simulink model "experiment_supervisor"  (R2023b)
settings: Solver=FixedStepDiscrete  StartTime=0.0  StopTime=inf  FixedStep=Ts  RelTol=1e-3
model workspace (MAT data in the model file):
  Ts = Simulink.Parameter
  Ts.Value = 0.01
  Ts.DataType = 'auto'
  Ts.DocUnits = 's'
  Ts.Complexity = 'real'
  Ts.Dimensions = [1 1]
  board_ID = Simulink.Parameter
  board_ID.Value = 1
  board_ID.DataType = 'auto'
  board_ID.Complexity = 'real'
  board_ID.Dimensions = [1 1]
undefined symbols (not defined in the file): CAN_ANGLE_DEG2ICUB, CAN_ANGLE_ICUB2DEG, CAN_VOLT_REF_SHIFT, canChannel
libraries: canmsglib x12, canlib x4, simulink x1, hdlsllib x1
settings Model: DataDictionary=EmbeddedBoardDD.sldd  Creator=upattacini  LastModifiedBy=mfussi
settings SolverCC: AlgebraicLoopSolver=TrustRegion  DecoupledContinuousIntegration=on  MinimalZcImpactIntegration=on
settings OptimizationCC: ReuseModelBlockBuffer=off  SimCompilerOptimization=on
settings DebuggingCC: ParameterPrecisionLossMsg=none  UnconnectedInputMsg=warning  UnconnectedOutputMsg=warning  UnconnectedLineMsg=warning  ArithmeticOperatorsInVariantConditions=warning
settings HardwareCC: ProdBitPerLong=64  ProdHWDeviceType=Intel->x86-64 (Linux 64)
settings ModelReferenceCC: EnableRefExpFcnMdlSchedulingChecks=on
settings SFSimCC: SimUseLocalCustomCode=off  CustomCodeUndefinedFunction=UseInterfaceOnly
settings RTWCC: Description=Simulink Desktop Real-Time  SystemTargetFile=sldrt.tlc  TemplateMakefile=sldrt.tmf  RTWUseLocalCustomCode=off  RTWCompilerOptimization=on  DLArmComputeVersion=19.05
settings CodeAppCC: MaxIdLength=95
settings SimulinkDesktopRealTimeCC: TargetLibSuffix=_sldrt.a  TargetPreCompLibLocation=C:\Program Files\MATLAB\R2023b\toolbox\sldrt\lib\win64

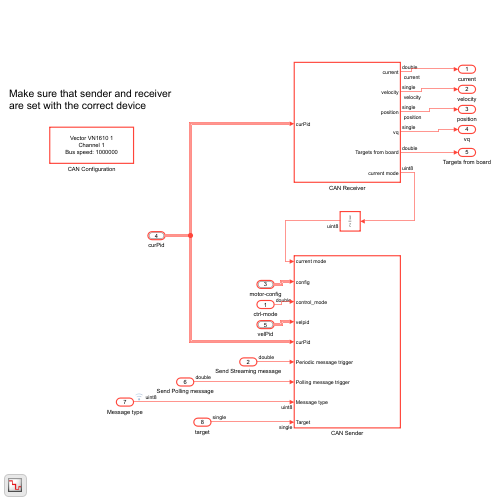
[thumbnail: Simulink's stored preview of the top-level diagram]
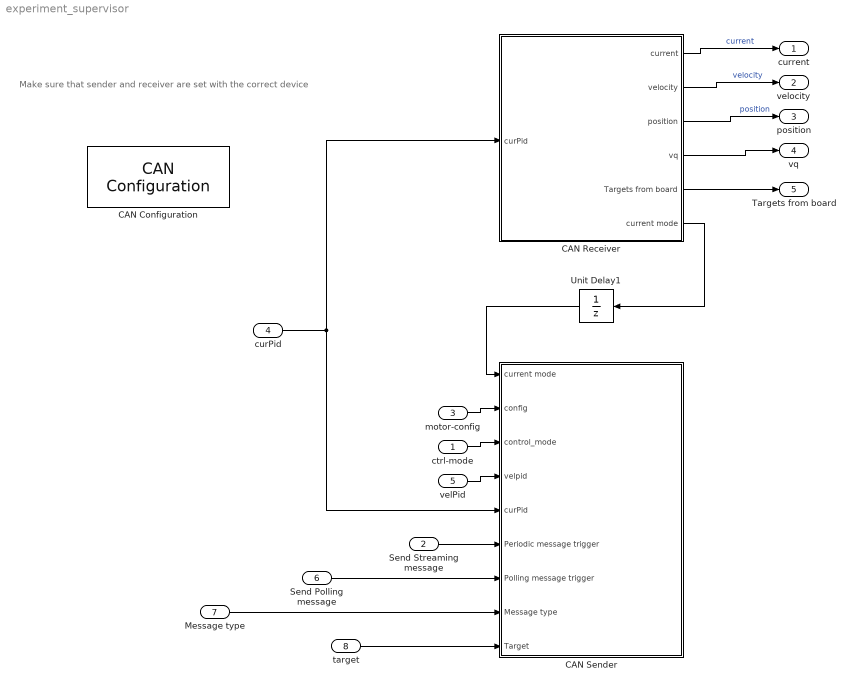
== system experiment_supervisor ==
  note: Make sure that sender and receiver
      | are set with the correct device
  ctrl-mode : Inport
  Send Streaming message : Inport  Port=2
  motor-config : Inport  Port=3  OutDataTypeStr=Bus: MotorConfig
  curPid : Inport  Port=4  OutDataTypeStr=Bus: PIDConfig
  velPid : Inport  Port=5  OutDataTypeStr=Bus: PIDConfig
  Send Polling message : Inport  Port=6
  Message type : Inport  Port=7
  target : Inport  Port=8  OutDataTypeStr=single
  CAN Configuration : canlib/CAN Configuration  BlockHandle=989.0002  Device=Vector VN1610 1 (Channel 1)  DeviceMenu=Vector VN1610 1 (Channel 1)  ObjConstructor=canChannel('Vector', 'VN1610 1', 1)  BusSpeed=1000000  EnableBitParameters=off  SJW=1  TSEG1=4  TSEG2=3  NSamples=1  AckMode=Normal
  CAN Receiver : Subsystem
  CAN Sender : Subsystem
  Unit Delay1 : UnitDelay  SampleTime=-1  HasFrameUpgradeWarning=on
  current : Outport
  velocity : Outport  Port=2
  position : Outport  Port=3
  vq : Outport  Port=4
  Targets from board : Outport  Port=5
  wires:
  CAN Receiver/6(current mode) -> Unit Delay1/1
  curPid/1 -> CAN Sender/5(curPid), CAN Receiver/1(curPid)
  CAN Receiver/5(Targets from board) -> Targets from board/1
  CAN Receiver/1(current) -> current/1  "current"
  CAN Receiver/4(vq) -> vq/1
  CAN Receiver/3(position) -> position/1  "position"
  CAN Receiver/2(velocity) -> velocity/1  "velocity"
  motor-config/1 -> CAN Sender/2(config)
  ctrl-mode/1 -> CAN Sender/3(control_mode)
  velPid/1 -> CAN Sender/4(velpid)
  Send Streaming message/1 -> CAN Sender/6(Periodic message trigger)
  Unit Delay1/1 -> CAN Sender/1(current mode)
  Send Polling message/1 -> CAN Sender/7(Polling message trigger)
  Message type/1 -> CAN Sender/8(Message type)
  target/1 -> CAN Sender/9(Target)

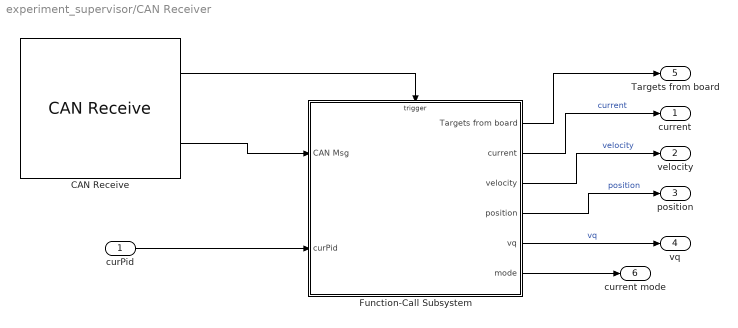
== system experiment_supervisor/CAN Receiver ==
  curPid : Inport  OutDataTypeStr=Bus: PIDConfig
  CAN Receive : canlib/CAN Receive  BlockHandle=992.0002  Device=Vector VN1610 1 (Channel 1)  DeviceMenu=Vector VN1610 1 (Channel 1)  ObjConstructor=canChannel('Vector', 'VN1610 1', 1)  EnableStandardIDsFilter=off  StdIDsCombo=Allow all  StandardIDs=0  EnableExtendedIDsFilter=off  ExtIDsCombo=Allow all  ExtendedIDs=0  SampleTime=Ts  MsgsPerTimestep=all  InternalFilterUpdateStatus=on  BusOutput=on
  Function-Call Subsystem : Subsystem  TreatAsAtomicUnit=on
  current : Outport
  velocity : Outport  Port=2
  position : Outport  Port=3
  vq : Outport  Port=4
  Targets from board : Outport  Port=5
  current mode : Outport  Port=6
  wires:
  CAN Receive/1 -> Function-Call Subsystem/Trigger
  CAN Receive/2 -> Function-Call Subsystem/1(CAN Msg)
  Function-Call Subsystem/2(current) -> current/1  "current"
  Function-Call Subsystem/3(velocity) -> velocity/1  "velocity"
  Function-Call Subsystem/4(position) -> position/1  "position"
  Function-Call Subsystem/5(vq) -> vq/1  "vq"
  Function-Call Subsystem/1(Targets from board) -> Targets from board/1
  curPid/1 -> Function-Call Subsystem/2(curPid)
  Function-Call Subsystem/6(mode) -> current mode/1

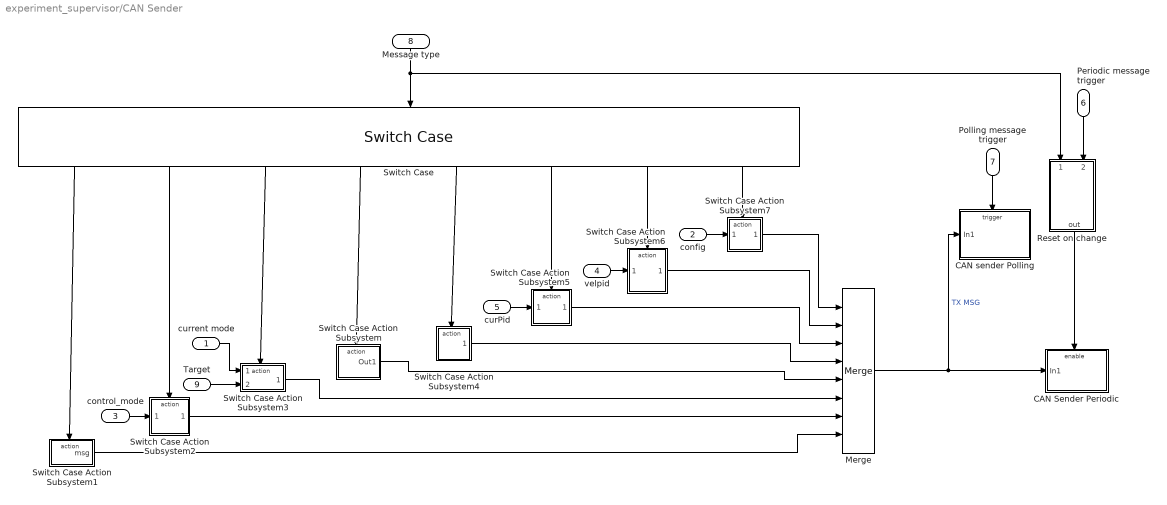
== system experiment_supervisor/CAN Sender ==
  current mode : Inport
  config : Inport  Port=2  OutDataTypeStr=Bus: MotorConfig
  control_mode : Inport  Port=3
  velpid : Inport  Port=4
  curPid : Inport  Port=5
  Periodic message trigger : Inport  Port=6
  Polling message trigger : Inport  Port=7
  Message type : Inport  Port=8  OutDataTypeStr=uint8
  Target : Inport  Port=9  OutDataTypeStr=single
  CAN Sender Periodic : Subsystem  TreatAsAtomicUnit=on
  CAN sender Polling : Subsystem
  Merge : Merge  Inputs=8
  Reset on change : Subsystem
  Switch Case : SwitchCase  CaseConditions={1,2,3,4,5,6,7,8}  ShowDefaultCase=off
  Switch Case Action Subsystem : Subsystem  TreatAsAtomicUnit=on
  Switch Case Action Subsystem1 : Subsystem  TreatAsAtomicUnit=on
  Switch Case Action Subsystem2 : Subsystem  TreatAsAtomicUnit=on
  Switch Case Action Subsystem3 : Subsystem  TreatAsAtomicUnit=on
  Switch Case Action Subsystem4 : Subsystem  TreatAsAtomicUnit=on
  Switch Case Action Subsystem5 : Subsystem  TreatAsAtomicUnit=on
  Switch Case Action Subsystem6 : Subsystem  TreatAsAtomicUnit=on
  Switch Case Action Subsystem7 : Subsystem  TreatAsAtomicUnit=on
  wires:
  Message type/1 -> Reset on change/1(message type), Switch Case/1
  Polling message trigger/1 -> CAN sender Polling/Trigger
  Merge/1 -> CAN Sender Periodic/1(In1), CAN sender Polling/1(In1)  "TX MSG"
  control_mode/1 -> Switch Case Action Subsystem2/1(control_mode)
  current mode/1 -> Switch Case Action Subsystem3/1(mode)
  Target/1 -> Switch Case Action Subsystem3/2(target)
  Switch Case/1 -> Switch Case Action Subsystem1/Action
  Switch Case/2 -> Switch Case Action Subsystem2/Action
  Switch Case/3 -> Switch Case Action Subsystem3/Action
  Switch Case/4 -> Switch Case Action Subsystem/Action
  Switch Case/5 -> Switch Case Action Subsystem4/Action
  Switch Case/6 -> Switch Case Action Subsystem5/Action
  Switch Case/7 -> Switch Case Action Subsystem6/Action
  Switch Case/8 -> Switch Case Action Subsystem7/Action
  config/1 -> Switch Case Action Subsystem7/1(cfg)
  Switch Case Action Subsystem7/1(Out1) -> Merge/1
  Switch Case Action Subsystem6/1(Out1) -> Merge/2
  Switch Case Action Subsystem5/1(" ") -> Merge/3
  Switch Case Action Subsystem4/1(Out1) -> Merge/4
  Switch Case Action Subsystem/1(Out1) -> Merge/5
  Switch Case Action Subsystem3/1(msg) -> Merge/6
  Switch Case Action Subsystem2/1(msg) -> Merge/7
  Switch Case Action Subsystem1/1(msg) -> Merge/8
  curPid/1 -> Switch Case Action Subsystem5/1(curPid)
  velpid/1 -> Switch Case Action Subsystem6/1(velPid1)
  Periodic message trigger/1 -> Reset on change/2(enable periodic)
  Reset on change/1(out) -> CAN Sender Periodic/Enable

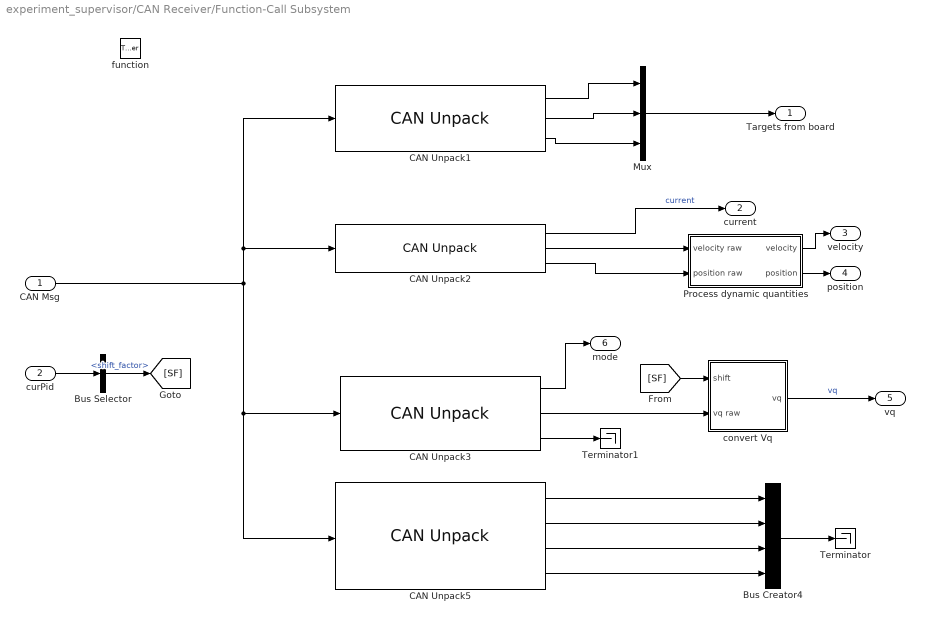
== system experiment_supervisor/CAN Receiver/Function-Call Subsystem ==
  CAN Msg : Inport
  curPid : Inport  Port=2  OutDataTypeStr=Bus: PIDConfig
  function : TriggerPort  TriggerType=function-call  VariantControl=(inherit)
  Bus Creator4 : BusCreator  Inputs=4
  Bus Selector : BusSelector  OutputSignals=shift_factor
  CAN Unpack1 : canmsglib/CAN Unpack  MsgList=(none)  MsgName=TARGETS  MsgIDType=Standard (11-bit identifier)  MsgIdentifier=0x10F  MsgLength=8  SignalInfo={ 'Target1', '0', '16', 'LE', 'signed', 'Standard', '0', '1', '0', '-Inf', 'Inf'; 'Target2', '16', '16', 'LE', 'signed', 'Standard', '0', '1', '0', '-Inf', 'Inf'; 'Target3', '32', '16', 'LE', 'signed', 'Standard', '0', '1', '0', '-Inf', 'Inf' }  IDPort=off  TimestampPort=off  ErrorPort=off  RemotePort=off  LengthPort=off  StatusPort=off  ApplyMinMax=off
  CAN Unpack2 : canmsglib/CAN Unpack  MsgList=(none)  MsgName=FOC  MsgIDType=Standard (11-bit identifier)  MsgIdentifier=0x110  MsgLength=8  SignalInfo={ 'current', '0', '16', 'LE', 'signed', 'Standard', '0', '1', '0', '-Inf', 'Inf'; 'velocity', '16', '16', 'LE', 'signed', 'Standard', '0', '1', '0', '-Inf', 'Inf'; 'position', '32', '32', 'LE', 'signed', 'Standard', '0', '1', '0', '-Inf', 'Inf' }  IDPort=off  TimestampPort=off  ErrorPort=off  RemotePort=off  LengthPort=off  StatusPort=off  ApplyMinMax=off
  CAN Unpack3 : canmsglib/CAN Unpack  MsgList=(none)  MsgName=STATUS  MsgIDType=Standard (11-bit identifier)  MsgIdentifier=0x113  MsgLength=8  SignalInfo={ 'mode', '0', '8', 'LE', 'unsigned', 'Standard', '0', '1', '0', '-Inf', 'Inf'; 'pwm', '16', '16', 'LE', 'signed', 'Standard', '0', '1', '0', '-Inf', 'Inf'; 'fault', '32', '8', 'LE', 'unsigned', 'Standard', '0', '1', '0', '-Inf', 'Inf' }  IDPort=off  TimestampPort=off  ErrorPort=off  RemotePort=off  LengthPort=off  StatusPort=off  ApplyMinMax=off
  CAN Unpack5 : canmsglib/CAN Unpack  MsgList=(none)  MsgName=DISCOVER  MsgIDType=Standard (11-bit identifier)  MsgIdentifier=0x710  MsgLength=5  SignalInfo={}  IDPort=on  TimestampPort=on  ErrorPort=off  RemotePort=off  LengthPort=on  StatusPort=off  ApplyMinMax=off
      settings: DataFormat=raw data
  Mux : Mux  Inputs=3
  Process dynamic quantities : Subsystem
  Terminator : Terminator
  Terminator1 : Terminator
  convert Vq : Subsystem
  Targets from board : Outport
  current : Outport  Port=2  Unit=mA
  velocity : Outport  Port=3
  position : Outport  Port=4
  vq : Outport  Port=5  PortDimensions=1
  mode : Outport  Port=6  OutDataTypeStr=uint8
  wires:
  CAN Unpack5/4 -> Bus Creator4/4
  CAN Unpack5/3 -> Bus Creator4/3
  CAN Unpack5/2 -> Bus Creator4/2
  CAN Unpack5/1 -> Bus Creator4/1
  Bus Creator4/1 -> Terminator/1
  CAN Unpack1/1 -> Mux/1
  CAN Unpack1/2 -> Mux/2
  CAN Unpack1/3 -> Mux/3
  Mux/1 -> Targets from board/1
  curPid/1 -> Bus Selector/1
  CAN Unpack2/2 -> Process dynamic quantities/1(velocity raw)
  CAN Unpack2/1 -> current/1  "current"
  Process dynamic quantities/2(position) -> position/1
  Process dynamic quantities/1(velocity) -> velocity/1
  CAN Unpack2/3 -> Process dynamic quantities/2(position raw)
  CAN Unpack3/2 -> convert Vq/2(vq raw)
  CAN Unpack3/1 -> mode/1
  convert Vq/1(vq) -> vq/1  "vq"
  CAN Msg/1 -> CAN Unpack2/1, CAN Unpack1/1, CAN Unpack5/1, CAN Unpack3/1
  CAN Unpack3/3 -> Terminator1/1
  Bus Selector/1 -> [SF]  "<shift_factor>"
  [SF] -> convert Vq/1(shift)

== system experiment_supervisor/CAN Sender/CAN Sender Periodic ==
  In1 : Inport
  Enable : EnablePort
  CAN Transmit : canlib/CAN Transmit  BlockHandle=1101.0002  Device=Vector VN1610 1 (Channel 1)  DeviceMenu=Vector VN1610 1 (Channel 1)  ObjConstructor=canChannel('Vector', 'VN1610 1', 1)  EnableEventTransmit=off  EnablePeriodicTransmit=on  MessagePeriod=Ts
  wires:
  In1/1 -> CAN Transmit/1

== system experiment_supervisor/CAN Sender/CAN sender Polling ==
  In1 : Inport
  Trigger : TriggerPort  VariantControl=(inherit)  PortDimensions=1
  CAN Transmit : canlib/CAN Transmit  BlockHandle=1106.0002  Device=Vector VN1610 1 (Channel 1)  DeviceMenu=Vector VN1610 1 (Channel 1)  ObjConstructor=canChannel('Vector', 'VN1610 1', 1)  EnableEventTransmit=off  EnablePeriodicTransmit=off  MessagePeriod=1.000
  wires:
  In1/1 -> CAN Transmit/1

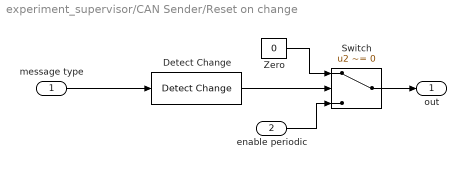
== system experiment_supervisor/CAN Sender/Reset on change ==
  message type : Inport
  enable periodic : Inport  Port=2
  Detect Change : simulink/Logic and Bit Operations/Detect Change  vinit=0  OutDataTypeStr=boolean
  Switch : Switch  Criteria=u2 ~= 0  SaturateOnIntegerOverflow=off  InputSameDT=off
  Zero : Constant  Value=0  OutDataTypeStr=Inherit: Inherit via back propagation
  out : Outport
  wires:
  Switch/1 -> out/1
  enable periodic/1 -> Switch/3
  Detect Change/1 -> Switch/2
  message type/1 -> Detect Change/1
  Zero/1 -> Switch/1

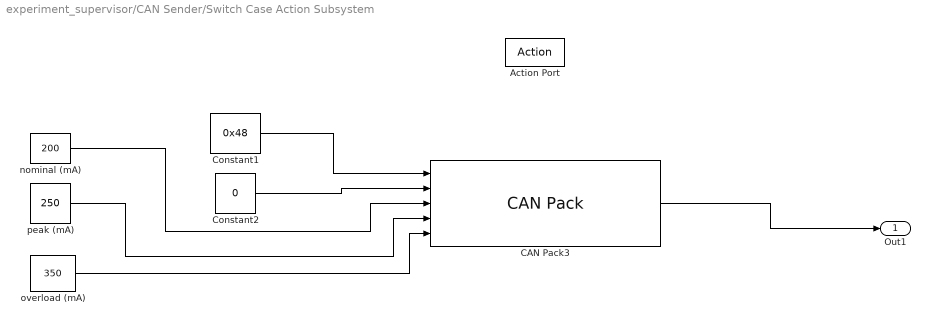
== system experiment_supervisor/CAN Sender/Switch Case Action Subsystem ==
  Action Port : ActionPort  ActionPortLabel=case [ 4 ]:
  CAN Pack3 : canmsglib/CAN Pack  MsgList=(none)  MsgName=CAN Limits  MsgIDType=Standard (11-bit identifier)  MsgIdentifier=board_ID  MsgLength=8  Remote=off  ApplyMinMax=off  BusOutput=on  SignalInfo={ 'CMD', '0', '8', 'LE', 'unsigned', 'Standard', '0', '1', '0', '-Inf', 'Inf'; 'X', '8', '8', 'LE', 'unsigned', 'Standard', '0', '1', '0', '-Inf', 'Inf'; 'NOMINAL', '16', '16', 'LE', 'unsigned', 'Standard', '0', '1', '0', '-Inf', 'Inf'; 'PEAK', '32', '16', 'LE', 'unsigned', 'Standard', '0', '1', '0', '-Inf', 'Inf'; 'OVERLOAD', '48', '16', 'LE', 'unsigned', 'Standard', '0', '1', '0', '-Inf', 'Inf' }
      settings: DataFormat=manually specified signals
  Constant1 : Constant  Value=0x48  OutDataTypeStr=Inherit: Inherit via back propagation
  Constant2 : Constant  Value=0  OutDataTypeStr=Inherit: Inherit via back propagation
  nominal (mA) : Constant  Value=200  OutDataTypeStr=Inherit: Inherit via back propagation
  overload (mA) : Constant  Value=350  OutDataTypeStr=Inherit: Inherit via back propagation
  peak (mA) : Constant  Value=250  OutDataTypeStr=Inherit: Inherit via back propagation
  Out1 : Outport
  wires:
  peak (mA)/1 -> CAN Pack3/4
  nominal (mA)/1 -> CAN Pack3/3
  overload (mA)/1 -> CAN Pack3/5
  Constant2/1 -> CAN Pack3/2
  Constant1/1 -> CAN Pack3/1
  CAN Pack3/1 -> Out1/1

== system experiment_supervisor/CAN Sender/Switch Case Action Subsystem1 ==
  Action Port : ActionPort  ActionPortLabel=case [ 1 ]:
  CAN Pack : canmsglib/CAN Pack  MsgList=(none)  MsgName=CAN Idle  MsgIDType=Standard (11-bit identifier)  MsgIdentifier=board_ID  MsgLength=2  Remote=off  ApplyMinMax=off  BusOutput=on  SignalInfo={ 'Idle', '0', '16', 'LE', 'unsigned', 'Standard', '0', '1', '0', '-Inf', 'Inf' }
      settings: DataFormat=manually specified signals
  idle-mode : Constant  Value=0x09  OutDataTypeStr=uint8
  msg : Outport
  wires:
  CAN Pack/1 -> msg/1
  idle-mode/1 -> CAN Pack/1

== system experiment_supervisor/CAN Sender/Switch Case Action Subsystem2 ==
  control_mode : Inport
  Action Port : ActionPort  ActionPortLabel=case [ 2 ]:
  CAN Pack1 : canmsglib/CAN Pack  MsgList=(none)  MsgName=SET Control Mode  MsgIDType=Standard (11-bit identifier)  MsgIdentifier=board_ID  MsgLength=2  Remote=off  ApplyMinMax=off  BusOutput=on  SignalInfo={ 'CMD', '0', '8', 'LE', 'unsigned', 'Standard', '0', '1', '0', '-Inf', 'Inf'; 'CTRL', '8', '8', 'LE', 'signed', 'Standard', '0', '1', '0', '-Inf', 'Inf' }
      settings: DataFormat=manually specified signals
  current-mode : Constant  Value=0x09  OutDataTypeStr=uint8
  msg : Outport
  wires:
  CAN Pack1/1 -> msg/1
  current-mode/1 -> CAN Pack1/1
  control_mode/1 -> CAN Pack1/2

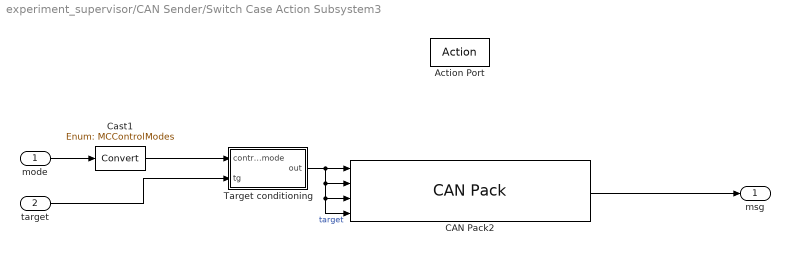
== system experiment_supervisor/CAN Sender/Switch Case Action Subsystem3 ==
  mode : Inport
  target : Inport  Port=2
  Action Port : ActionPort  ActionPortLabel=case [ 3 ]:
  CAN Pack2 : canmsglib/CAN Pack  MsgList=(none)  MsgName=CAN Target  MsgIDType=Standard (11-bit identifier)  MsgIdentifier=0x10F  MsgLength=8  Remote=off  ApplyMinMax=off  BusOutput=on  SignalInfo={ 'Target 1', '0', '16', 'LE', 'signed', 'Standard', '0', '1', '0', '-Inf', 'Inf'; 'Target 2', '16', '16', 'LE', 'signed', 'Standard', '0', '1', '0', '-Inf', 'Inf'; 'Target 3', '32', '16', 'LE', 'signed', 'Standard', '0', '1', '0', '-Inf', 'Inf'; 'Target 4', '48', '16', 'LE', 'signed', 'Standard', '0', '1', '0', '-Inf', 'Inf' }
      settings: DataFormat=manually specified signals
  Cast1 : DataTypeConversion  OutDataTypeStr=Enum: MCControlModes  SaturateOnIntegerOverflow=off  RndMeth=Floor
  Target conditioning : Subsystem
  msg : Outport
  wires:
  CAN Pack2/1 -> msg/1
  Cast1/1 -> Target conditioning/1(control_mode)
  Target conditioning/1(out) -> CAN Pack2/4, CAN Pack2/3, CAN Pack2/2, CAN Pack2/1  "target"
  target/1 -> Target conditioning/2(tg)
  mode/1 -> Cast1/1

== system experiment_supervisor/CAN Sender/Switch Case Action Subsystem4 ==
  Action Port : ActionPort  ActionPortLabel=case [ 5 ]:
  CAN Pack4 : canmsglib/CAN Pack  MsgList=(none)  MsgName=DISCOVER  MsgIDType=Standard (11-bit identifier)  MsgIdentifier=0x70F  MsgLength=1  Remote=off  ApplyMinMax=off  BusOutput=on  SignalInfo={}
      settings: DataFormat=raw data
  discover : Constant  Value=0xFF
  Out1 : Outport
  wires:
  CAN Pack4/1 -> Out1/1
  discover/1 -> CAN Pack4/1

== system experiment_supervisor/CAN Sender/Switch Case Action Subsystem5 ==
  curPid : Inport
  Action Port : ActionPort  ActionPortLabel=case [ 6 ]:
  Bus Selector1 : BusSelector  OutputSignals=P,I,D,shift_factor
  CAN Pack5 : canmsglib/CAN Pack  MsgList=(none)  MsgName=SET_CURRENT_PID  MsgIDType=Standard (11-bit identifier)  MsgIdentifier=board_ID  MsgLength=8  Remote=off  ApplyMinMax=off  BusOutput=on  SignalInfo={ 'CMD', '0', '8', 'LE', 'unsigned', 'Standard', '0', '1', '0', '-Inf', 'Inf'; 'Kp', '8', '16', 'LE', 'signed', 'Standard', '0', '1', '0', '-Inf', 'Inf'; 'Ki', '24', '16', 'LE', 'signed', 'Standard', '0', '1', '0', '-Inf', 'Inf'; 'Kd', '40', '16', 'LE', 'signed', 'Standard', '0', '1', '0', '-Inf', 'Inf'; 'shift', '56', '8', 'LE', 'unsigned', 'Standard', '0', '1', '0', '-Inf', 'Inf' }
      settings: DataFormat=manually specified signals
  current pid : Constant  Value=0x65  OutDataTypeStr=int16
  " " : Outport
  wires:
  curPid/1 -> Bus Selector1/1
  Bus Selector1/3 -> CAN Pack5/4  "<D>"
  Bus Selector1/2 -> CAN Pack5/3  "<I>"
  CAN Pack5/1 -> " "/1
  current pid/1 -> CAN Pack5/1
  Bus Selector1/1 -> CAN Pack5/2  "<P>"
  Bus Selector1/4 -> CAN Pack5/5  "<shift_factor>"

== system experiment_supervisor/CAN Sender/Switch Case Action Subsystem6 ==
  velPid1 : Inport  OutDataTypeStr=Bus: PIDConfig
  Action Port : ActionPort  ActionPortLabel=case [ 7 ]:
  Bus Selector : BusSelector  OutputSignals=P,I,D,shift_factor
  CAN Pack6 : canmsglib/CAN Pack  MsgList=(none)  MsgName=SET_VELOCITY_PID  MsgIDType=Standard (11-bit identifier)  MsgIdentifier=board_ID  MsgLength=8  Remote=off  ApplyMinMax=off  BusOutput=on  SignalInfo={ 'CMD', '0', '8', 'LE', 'unsigned', 'Standard', '0', '1', '0', '-Inf', 'Inf'; 'Kp', '8', '16', 'LE', 'signed', 'Standard', '0', '1', '0', '-Inf', 'Inf'; 'Ki', '24', '16', 'LE', 'signed', 'Standard', '0', '1', '0', '-Inf', 'Inf'; 'Kd', '40', '16', 'LE', 'signed', 'Standard', '0', '1', '0', '-Inf', 'Inf'; 'shift', '56', '8', 'LE', 'unsigned', 'Standard', '0', '1', '0', '-Inf', 'Inf' }
      settings: DataFormat=manually specified signals
  velocity pid : Constant  Value=0x69  OutDataTypeStr=int16
  Out1 : Outport
  wires:
  CAN Pack6/1 -> Out1/1
  Bus Selector/3 -> CAN Pack6/4  "<D>"
  Bus Selector/4 -> CAN Pack6/5  "<shift_factor>"
  velPid1/1 -> Bus Selector/1
  Bus Selector/2 -> CAN Pack6/3  "<I>"
  Bus Selector/1 -> CAN Pack6/2  "<P>"
  velocity pid/1 -> CAN Pack6/1

== system experiment_supervisor/CAN Sender/Switch Case Action Subsystem7 ==
  cfg : Inport
  Action Port : ActionPort  ActionPortLabel=case [ 8 ]:
  CAN Pack5 : canmsglib/CAN Pack  MsgList=(none)  MsgName=Set_Motor_Config  MsgIDType=Standard (11-bit identifier)  MsgIdentifier=board_ID  MsgLength=8  Remote=off  ApplyMinMax=off  BusOutput=on  SignalInfo={ 'CMD', '0', '8', 'LE', 'unsigned', 'Standard', '0', '1', '0', '-Inf', 'Inf'; 'FLAGS', '8', '8', 'LE', 'unsigned', 'Standard', '0', '1', '0', '-Inf', 'Inf'; 'RES_ENCODER', '16', '16', 'LE', 'signed', 'Standard', '0', '1', '0', '-Inf', 'Inf'; 'OFFSET_ENCODER', '32', '16', 'LE', 'unsigned', 'Standard', '0', '1', '0', '-Inf', 'Inf'; 'N_POLES', '48', '8', 'LE', 'unsigned', 'Standard', '0', '1', '0', '-Inf', 'Inf'; 'ENCODER_TOLERANCE', '56', '8', 'LE', 'unsigned', 'Standard', '0', '1', '0', '-Inf', 'Inf' }
      settings: DataFormat=manually specified signals
  Constant3 : Constant  Value=0x77  OutDataTypeStr=Inherit: Inherit via back propagation
  Unpack motor configuration : MATLAB Function  TreatAsAtomicUnit=on
  Out1 : Outport
  wires:
  Unpack motor configuration/5(enc_tolerance) -> CAN Pack5/6
  Unpack motor configuration/2(resolution) -> CAN Pack5/3
  cfg/1 -> Unpack motor configuration/1(motor_cfg)
  Unpack motor configuration/3(rotor_offset) -> CAN Pack5/4
  Unpack motor configuration/4(n_poles) -> CAN Pack5/5
  Unpack motor configuration/1(flags) -> CAN Pack5/2
  Constant3/1 -> CAN Pack5/1
  CAN Pack5/1 -> Out1/1

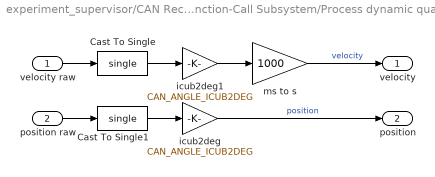
== system experiment_supervisor/CAN Receiver/Function-Call Subsystem/Process dynamic quantities ==
  velocity raw : Inport
  position raw : Inport  Port=2
  Cast To Single : DataTypeConversion  OutDataTypeStr=single  SaturateOnIntegerOverflow=off  RndMeth=Floor
  Cast To Single1 : DataTypeConversion  OutDataTypeStr=single  SaturateOnIntegerOverflow=off  RndMeth=Floor
  icub2deg : Gain  Gain=CAN_ANGLE_ICUB2DEG
  icub2deg1 : Gain  Gain=CAN_ANGLE_ICUB2DEG
  ms to s : Gain  Gain=1000
  velocity : Outport
  position : Outport  Port=2
  wires:
  Cast To Single1/1 -> icub2deg/1
  icub2deg1/1 -> ms to s/1
  Cast To Single/1 -> icub2deg1/1
  icub2deg/1 -> position/1  "position"
  velocity raw/1 -> Cast To Single/1
  position raw/1 -> Cast To Single1/1
  ms to s/1 -> velocity/1  "velocity"

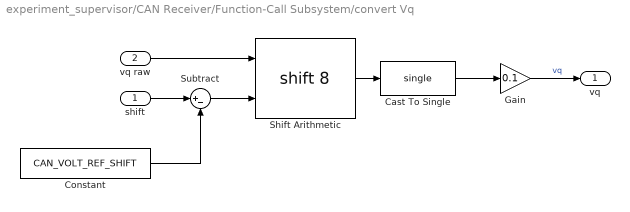
== system experiment_supervisor/CAN Receiver/Function-Call Subsystem/convert Vq ==
  shift : Inport
  vq raw : Inport  Port=2
  Cast To Single : DataTypeConversion  OutDataTypeStr=single  SaturateOnIntegerOverflow=off  RndMeth=Floor
  Constant : Constant  Value=CAN_VOLT_REF_SHIFT
  Gain : Gain  Gain=0.1
  Shift Arithmetic : ArithShift  BitShiftNumberSource=Input port  BitShiftNumber=8
      settings: InputPortMap=u0,p1
  Subtract : Sum  Inputs=|+-
  vq : Outport
  wires:
  Shift Arithmetic/1 -> Cast To Single/1
  vq raw/1 -> Shift Arithmetic/1
  Cast To Single/1 -> Gain/1
  Gain/1 -> vq/1  "vq"
  shift/1 -> Subtract/1
  Constant/1 -> Subtract/2
  Subtract/1 -> Shift Arithmetic/2

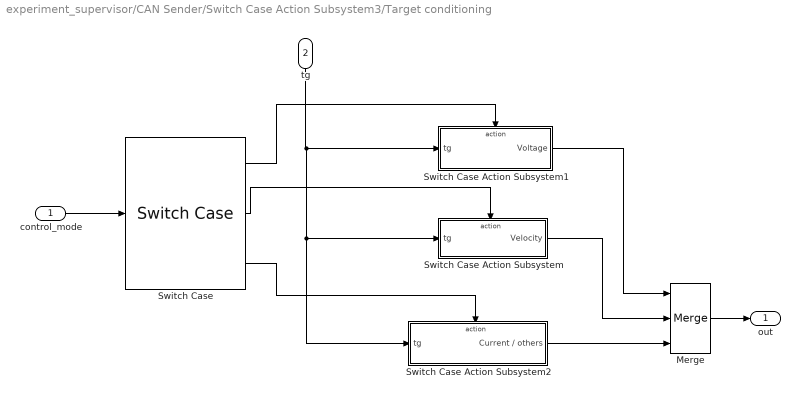
== system experiment_supervisor/CAN Sender/Switch Case Action Subsystem3/Target conditioning ==
  control_mode : Inport
  tg : Inport  Port=2
  Merge : Merge  Inputs=3  InitialOutput=0
  Switch Case : SwitchCase  CaseConditions={MCControlModes.OpenLoop, MCControlModes.SpeedVoltage}
  Switch Case Action Subsystem : Subsystem  TreatAsAtomicUnit=on
  Switch Case Action Subsystem1 : Subsystem  TreatAsAtomicUnit=on
  Switch Case Action Subsystem2 : Subsystem  TreatAsAtomicUnit=on
  out : Outport
  wires:
  tg/1 -> Switch Case Action Subsystem2/1(tg), Switch Case Action Subsystem/1(tg), Switch Case Action Subsystem1/1(tg)
  Switch Case/1 -> Switch Case Action Subsystem1/Action
  Switch Case/2 -> Switch Case Action Subsystem/Action
  Switch Case/3 -> Switch Case Action Subsystem2/Action
  Merge/1 -> out/1
  control_mode/1 -> Switch Case/1
  Switch Case Action Subsystem1/1(Voltage) -> Merge/1
  Switch Case Action Subsystem/1(Velocity) -> Merge/2
  Switch Case Action Subsystem2/1(Current / others) -> Merge/3

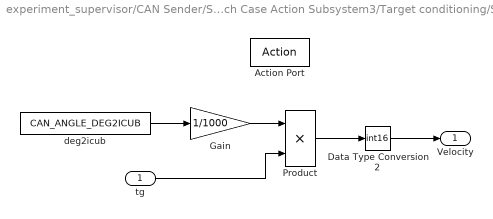
== system experiment_supervisor/CAN Sender/Switch Case Action Subsystem3/Target conditioning/Switch Case Action Subsystem ==
  tg : Inport
  Action Port : ActionPort  ActionPortLabel=case [ SpeedVoltage ]:
  Data Type Conversion2 : DataTypeConversion  OutDataTypeStr=int16  SaturateOnIntegerOverflow=off  RndMeth=Floor
  Gain : Gain  Gain=1/1000
  Product : Product
  deg2icub : Constant  Value=CAN_ANGLE_DEG2ICUB  OutDataTypeStr=single
  Velocity : Outport
  wires:
  tg/1 -> Product/2
  Gain/1 -> Product/1
  deg2icub/1 -> Gain/1
  Product/1 -> Data Type Conversion2/1
  Data Type Conversion2/1 -> Velocity/1

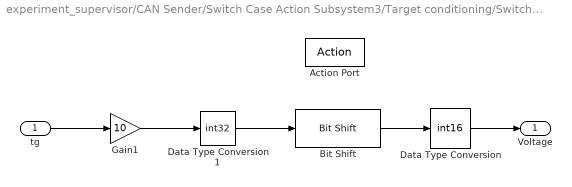
== system experiment_supervisor/CAN Sender/Switch Case Action Subsystem3/Target conditioning/Switch Case Action Subsystem1 ==
  tg : Inport
  Action Port : ActionPort  ActionPortLabel=case [ OpenLoop ]:
  Bit Shift : hdlsllib/Logic and Bit Operations/Bit Shift  mode=Shift Left Logical  N=5
  Data Type Conversion : DataTypeConversion  OutDataTypeStr=int16  SaturateOnIntegerOverflow=off  RndMeth=Floor
  Data Type Conversion1 : DataTypeConversion  OutDataTypeStr=int32  SaturateOnIntegerOverflow=off  RndMeth=Floor
  Gain1 : Gain  Gain=10
  Voltage : Outport
  wires:
  Bit Shift/1 -> Data Type Conversion/1
  Gain1/1 -> Data Type Conversion1/1
  tg/1 -> Gain1/1
  Data Type Conversion/1 -> Voltage/1
  Data Type Conversion1/1 -> Bit Shift/1

== system experiment_supervisor/CAN Sender/Switch Case Action Subsystem3/Target conditioning/Switch Case Action Subsystem2 ==
  tg : Inport
  Action Port : ActionPort  ActionPortLabel=default:
  Data Type Conversion3 : DataTypeConversion  OutDataTypeStr=int16  SaturateOnIntegerOverflow=off  RndMeth=Floor
  Current / others : Outport
  wires:
  tg/1 -> Data Type Conversion3/1
  Data Type Conversion3/1 -> Current / others/1

== matlab function experiment_supervisor/CAN Sender/Switch Case Action Subsystem7/Unpack motor configuration ==
  data: flags output; resolution output; rotor_offset output; n_poles output; motor_cfg input; enc_tolerance output
function [flags, resolution,rotor_offset, n_poles, enc_tolerance] = unpack_cfg(motor_cfg)

    flags = uint8(motor_cfg.has_quadrature_encoder); 
    flags = bitor(flags, bitshift(uint8(motor_cfg.has_hall_sens), 1));
    resolution = motor_cfg.rotor_encoder_resolution;
    rotor_offset = motor_cfg.rotor_index_offset;
    n_poles = motor_cfg.pole_pairs * 2;
    enc_tolerance = motor_cfg.encoder_tolerance;

end
